simulink model "PassStFwdBkwdCtrl"  (R2018b)
settings: Solver=FixedStepDiscrete  StartTime=0.0  StopTime=10.0  RelTol=1e-3
undefined symbols (not defined in the file or in its folder): KeSMSuMdMotFinshdTm_Val, KeSMSuMdRetryTm1_Val, KeSMSuModeReqDurgTm_Val
libraries: StCtrlLibBkRecln x1
settings Model: ModifiedHistory=2024.6.26 557模式流程V1.6  Creator=sn2xws  LastModifiedBy=sn2xws
settings DataIOCC: SaveFormat=StructureWithTime
settings OptimizationCC: DefaultParameterBehavior=Inlined  EnhancedBackFolding=on  PassReuseOutputArgsAs=Individual arguments  ZeroExternalMemoryAtStartup=off  ZeroInternalMemoryAtStartup=off  OptimizeBlockOrder=speed  DifferentSizesBufferReuse=on  OptimizationCustomize=off
settings DebuggingCC: ParameterTunabilityLossMsg=error
settings SFSimCC: MATLABDynamicMemAlloc=off
settings RTWCC: SystemTargetFile=autosar.tlc  GenCodeOnly=on  TemplateMakefile=ert_default_tmf  Description=AUTOSAR  GenerateReport=on  IncludeHyperlinkInReport=on  LaunchReport=on  GenerateTraceInfo=on  GenerateTraceReport=on  GenerateTraceReportSl=on  GenerateTraceReportSf=on  GenerateTraceReportEml=on
settings CodeAppCC: ForceParamTrailComments=on  IgnoreCustomStorageClasses=off  OperatorAnnotations=on  SimulinkDataObjDesc=on  SFDataObjDesc=on  InsertBlockDesc=on
settings STFCustomTargetCC: TargetLangStandard=C99 (ISO)  MultiwordLength=256  ParMdlRefBuildCompliant=on  CompOptLevelCompliant=on  IncludeMdlTerminateFcn=off  CombineOutputUpdateFcns=on  SuppressErrorStatus=on  ERTCustomFileBanners=on  SupportNonFinite=off  SupportComplex=off  SupportContinuousTime=off  SupportNonInlinedSFcns=off  RemoveResetFunc=on  MATLABClassNameForMDSCustomization=Simulink.SoftwareTarget.ERTCustomization  AutosarCompliant=on  UseToolchainInfoCompliant=on  LookupTableObjectStructAxisOrder=2,1,3,4,...  LUTObjectStructOrderEvenSpacing=Size,Table,Breakpoints  SystemTargetFile=autosar.tlc
settings ERTTargetCC: TargetLangStandard=C99 (ISO)  ConcurrentExecutionCompliant=off  IncludeMdlTerminateFcn=off  SuppressErrorStatus=on  SupportNonFinite=off  SupportComplex=off  ModelStepFunctionPrototypeControlCompliant=off  CPPClassGenCompliant=off  AutosarCompliant=on  LookupTableObjectStructAxisOrder=2,1,3,4,...  LUTObjectStructOrderEvenSpacing=Size,Table,Breakpoints  InlinedParameterPlacement=NonHierarchical  ERTCustomFileTemplate=example_file_process.tlc  ERTFilePackagingFormat=Compact

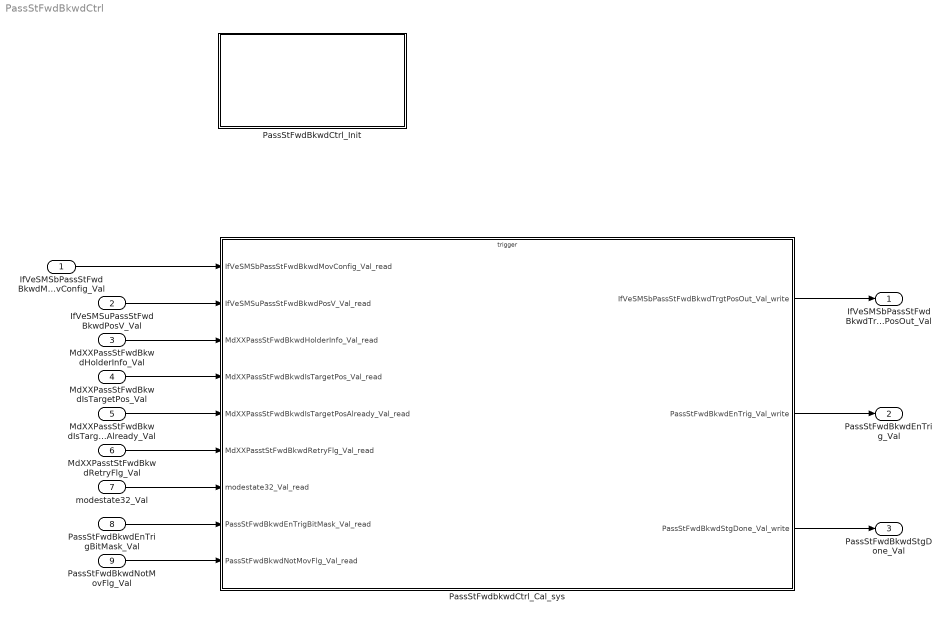
== system PassStFwdBkwdCtrl ==
  IfVeSMSbPassStFwdBkwdMovConfig_Val : Inport  OutDataTypeStr=boolean  PortDimensions=1
  IfVeSMSuPassStFwdBkwdPosV_Val : Inport  Port=2  OutDataTypeStr=boolean  PortDimensions=1
  MdXXPassStFwdBkwdHolderInfo_Val : Inport  Port=3  OutDataTypeStr=uint32  PortDimensions=1
  MdXXPassStFwdBkwdIsTargetPos_Val : Inport  Port=4  OutDataTypeStr=uint32  PortDimensions=1
  MdXXPassStFwdBkwdIsTargetPosAlready_Val : Inport  Port=5  OutDataTypeStr=uint32  PortDimensions=1
  MdXXPasstStFwdBkwdRetryFlg_Val : Inport  Port=6  OutDataTypeStr=uint32  PortDimensions=1
  modestate32_Val : Inport  Port=7  OutDataTypeStr=uint32  PortDimensions=1
  PassStFwdBkwdEnTrigBitMask_Val : Inport  Port=8  OutDataTypeStr=uint32  PortDimensions=1
  PassStFwdBkwdNotMovFlg_Val : Inport  Port=9  OutDataTypeStr=boolean  PortDimensions=1
  PassStFwdBkwdCtrl_Init : Subsystem
  PassStFwdbkwdCtrl_Cal_sys : Subsystem
  IfVeSMSbPassStFwdBkwdTrgtPosOut_Val : Outport  OutDataTypeStr=boolean  PortDimensions=1
  PassStFwdBkwdEnTrig_Val : Outport  Port=2  OutDataTypeStr=boolean  PortDimensions=1
  PassStFwdBkwdStgDone_Val : Outport  Port=3  OutDataTypeStr=boolean  PortDimensions=1
  wires:
  IfVeSMSbPassStFwdBkwdMovConfig_Val/1 -> PassStFwdbkwdCtrl_Cal_sys/1(IfVeSMSbPassStFwdBkwdMovConfig_Val_read)
  IfVeSMSuPassStFwdBkwdPosV_Val/1 -> PassStFwdbkwdCtrl_Cal_sys/2(IfVeSMSuPassStFwdBkwdPosV_Val_read)
  MdXXPassStFwdBkwdHolderInfo_Val/1 -> PassStFwdbkwdCtrl_Cal_sys/3(MdXXPassStFwdBkwdHolderInfo_Val_read)
  MdXXPassStFwdBkwdIsTargetPos_Val/1 -> PassStFwdbkwdCtrl_Cal_sys/4(MdXXPassStFwdBkwdIsTargetPos_Val_read)
  MdXXPassStFwdBkwdIsTargetPosAlready_Val/1 -> PassStFwdbkwdCtrl_Cal_sys/5(MdXXPassStFwdBkwdIsTargetPosAlready_Val_read)
  MdXXPasstStFwdBkwdRetryFlg_Val/1 -> PassStFwdbkwdCtrl_Cal_sys/6(MdXXPasstStFwdBkwdRetryFlg_Val_read)
  modestate32_Val/1 -> PassStFwdbkwdCtrl_Cal_sys/7(modestate32_Val_read)
  PassStFwdBkwdEnTrigBitMask_Val/1 -> PassStFwdbkwdCtrl_Cal_sys/8(PassStFwdBkwdEnTrigBitMask_Val_read)
  PassStFwdBkwdNotMovFlg_Val/1 -> PassStFwdbkwdCtrl_Cal_sys/9(PassStFwdBkwdNotMovFlg_Val_read)
  PassStFwdbkwdCtrl_Cal_sys/1(IfVeSMSbPassStFwdBkwdTrgtPosOut_Val_write) -> IfVeSMSbPassStFwdBkwdTrgtPosOut_Val/1
  PassStFwdbkwdCtrl_Cal_sys/2(PassStFwdBkwdEnTrig_Val_write) -> PassStFwdBkwdEnTrig_Val/1
  PassStFwdbkwdCtrl_Cal_sys/3(PassStFwdBkwdStgDone_Val_write) -> PassStFwdBkwdStgDone_Val/1

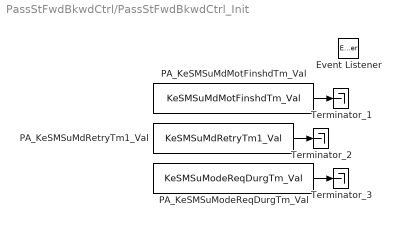
== system PassStFwdBkwdCtrl/PassStFwdBkwdCtrl_Init ==
  Event Listener : EventListener  EventName=reset
  PA_KeSMSuMdMotFinshdTm_Val : Constant  Value=KeSMSuMdMotFinshdTm_Val
  PA_KeSMSuMdRetryTm1_Val : Constant  Value=KeSMSuMdRetryTm1_Val
  PA_KeSMSuModeReqDurgTm_Val : Constant  Value=KeSMSuModeReqDurgTm_Val
  Terminator_1 : Terminator
  Terminator_2 : Terminator
  Terminator_3 : Terminator
  wires:
  PA_KeSMSuMdMotFinshdTm_Val/1 -> Terminator_1/1
  PA_KeSMSuMdRetryTm1_Val/1 -> Terminator_2/1
  PA_KeSMSuModeReqDurgTm_Val/1 -> Terminator_3/1

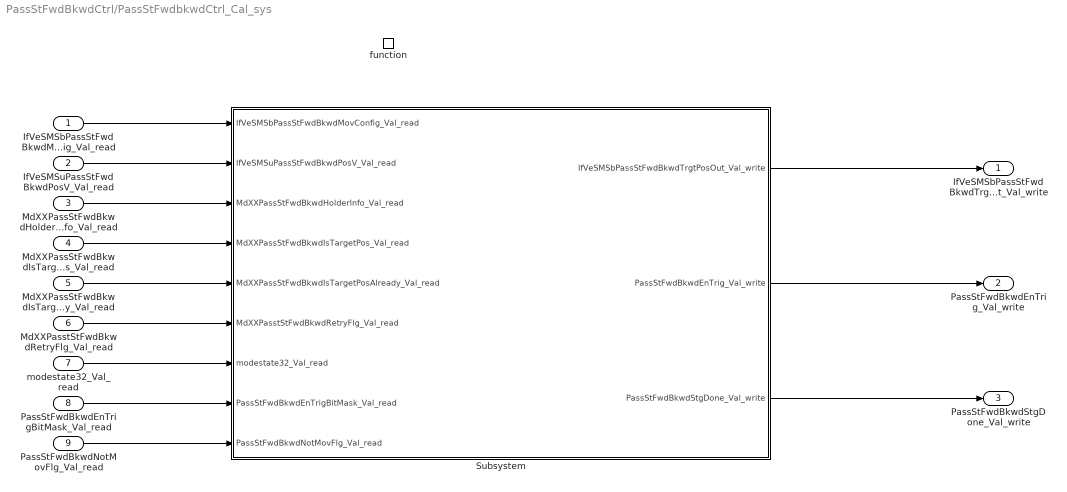
== system PassStFwdBkwdCtrl/PassStFwdbkwdCtrl_Cal_sys ==
  IfVeSMSbPassStFwdBkwdMovConfig_Val_read : Inport
  IfVeSMSuPassStFwdBkwdPosV_Val_read : Inport  Port=2
  MdXXPassStFwdBkwdHolderInfo_Val_read : Inport  Port=3
  MdXXPassStFwdBkwdIsTargetPos_Val_read : Inport  Port=4
  MdXXPassStFwdBkwdIsTargetPosAlready_Val_read : Inport  Port=5
  MdXXPasstStFwdBkwdRetryFlg_Val_read : Inport  Port=6
  modestate32_Val_read : Inport  Port=7
  PassStFwdBkwdEnTrigBitMask_Val_read : Inport  Port=8
  PassStFwdBkwdNotMovFlg_Val_read : Inport  Port=9
  function : TriggerPort  TriggerType=function-call  IsSimulinkFunction=on  FunctionName=PassStFwdbkwdCtrl_Cal  VariantControl=(inherit)
  Subsystem : Subsystem
  IfVeSMSbPassStFwdBkwdTrgtPosOut_Val_write : Outport
      settings: EnsureOutportIsVirtual=on
  PassStFwdBkwdEnTrig_Val_write : Outport  Port=2
      settings: EnsureOutportIsVirtual=on
  PassStFwdBkwdStgDone_Val_write : Outport  Port=3
      settings: EnsureOutportIsVirtual=on
  wires:
  IfVeSMSbPassStFwdBkwdMovConfig_Val_read/1 -> Subsystem/1(IfVeSMSbPassStFwdBkwdMovConfig_Val_read)
  IfVeSMSuPassStFwdBkwdPosV_Val_read/1 -> Subsystem/2(IfVeSMSuPassStFwdBkwdPosV_Val_read)
  MdXXPassStFwdBkwdHolderInfo_Val_read/1 -> Subsystem/3(MdXXPassStFwdBkwdHolderInfo_Val_read)
  MdXXPassStFwdBkwdIsTargetPos_Val_read/1 -> Subsystem/4(MdXXPassStFwdBkwdIsTargetPos_Val_read)
  MdXXPassStFwdBkwdIsTargetPosAlready_Val_read/1 -> Subsystem/5(MdXXPassStFwdBkwdIsTargetPosAlready_Val_read)
  MdXXPasstStFwdBkwdRetryFlg_Val_read/1 -> Subsystem/6(MdXXPasstStFwdBkwdRetryFlg_Val_read)
  modestate32_Val_read/1 -> Subsystem/7(modestate32_Val_read)
  PassStFwdBkwdEnTrigBitMask_Val_read/1 -> Subsystem/8(PassStFwdBkwdEnTrigBitMask_Val_read)
  PassStFwdBkwdNotMovFlg_Val_read/1 -> Subsystem/9(PassStFwdBkwdNotMovFlg_Val_read)
  Subsystem/1(IfVeSMSbPassStFwdBkwdTrgtPosOut_Val_write) -> IfVeSMSbPassStFwdBkwdTrgtPosOut_Val_write/1
  Subsystem/2(PassStFwdBkwdEnTrig_Val_write) -> PassStFwdBkwdEnTrig_Val_write/1
  Subsystem/3(PassStFwdBkwdStgDone_Val_write) -> PassStFwdBkwdStgDone_Val_write/1

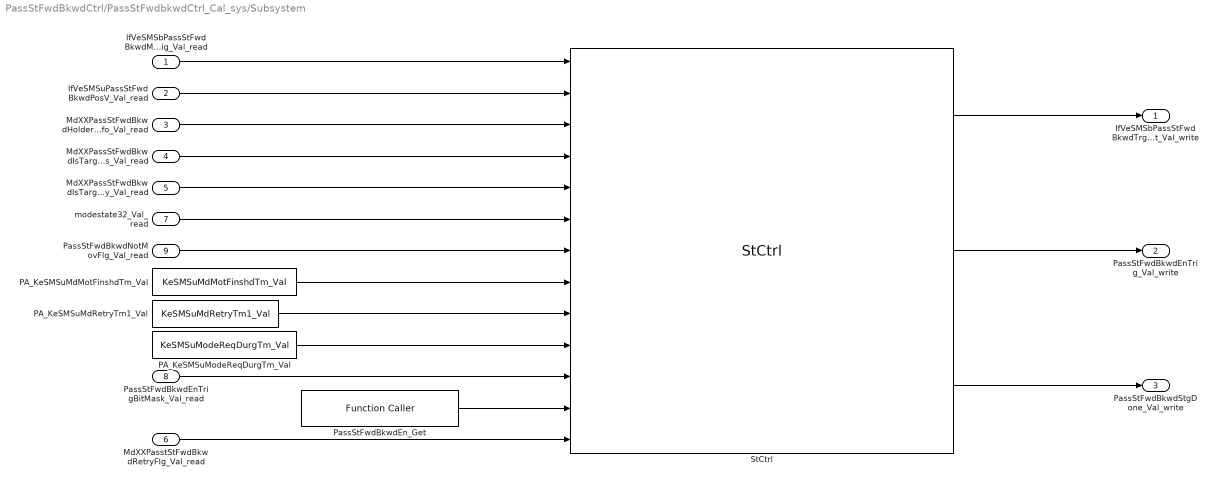
== system PassStFwdBkwdCtrl/PassStFwdbkwdCtrl_Cal_sys/Subsystem ==
  IfVeSMSbPassStFwdBkwdMovConfig_Val_read : Inport
  IfVeSMSuPassStFwdBkwdPosV_Val_read : Inport  Port=2
  MdXXPassStFwdBkwdHolderInfo_Val_read : Inport  Port=3
  MdXXPassStFwdBkwdIsTargetPos_Val_read : Inport  Port=4
  MdXXPassStFwdBkwdIsTargetPosAlready_Val_read : Inport  Port=5
  MdXXPasstStFwdBkwdRetryFlg_Val_read : Inport  Port=6
  modestate32_Val_read : Inport  Port=7
  PassStFwdBkwdEnTrigBitMask_Val_read : Inport  Port=8
  PassStFwdBkwdNotMovFlg_Val_read : Inport  Port=9
  PA_KeSMSuMdMotFinshdTm_Val : Constant  Value=KeSMSuMdMotFinshdTm_Val
  PA_KeSMSuMdRetryTm1_Val : Constant  Value=KeSMSuMdRetryTm1_Val
  PA_KeSMSuModeReqDurgTm_Val : Constant  Value=KeSMSuModeReqDurgTm_Val
  PassStFwdBkwdEn_Get : FunctionCaller  FunctionPrototype=data = PassStFwdBkwdEn_Get()  OutputArgumentSpecifications=uint32(1)
  StCtrl : StCtrlLibBkRecln/StCtrl  SystemSampleTime=-1
  IfVeSMSbPassStFwdBkwdTrgtPosOut_Val_write : Outport
      settings: EnsureOutportIsVirtual=on
  PassStFwdBkwdEnTrig_Val_write : Outport  Port=2
      settings: EnsureOutportIsVirtual=on
  PassStFwdBkwdStgDone_Val_write : Outport  Port=3
      settings: EnsureOutportIsVirtual=on
  wires:
  PA_KeSMSuModeReqDurgTm_Val/1 -> StCtrl/10
  PassStFwdBkwdEn_Get/1 -> StCtrl/12
  StCtrl/3 -> PassStFwdBkwdStgDone_Val_write/1
  StCtrl/2 -> PassStFwdBkwdEnTrig_Val_write/1
  StCtrl/1 -> IfVeSMSbPassStFwdBkwdTrgtPosOut_Val_write/1
  IfVeSMSbPassStFwdBkwdMovConfig_Val_read/1 -> StCtrl/1
  IfVeSMSuPassStFwdBkwdPosV_Val_read/1 -> StCtrl/2
  MdXXPassStFwdBkwdHolderInfo_Val_read/1 -> StCtrl/3
  MdXXPassStFwdBkwdIsTargetPos_Val_read/1 -> StCtrl/4
  MdXXPassStFwdBkwdIsTargetPosAlready_Val_read/1 -> StCtrl/5
  modestate32_Val_read/1 -> StCtrl/6
  PassStFwdBkwdNotMovFlg_Val_read/1 -> StCtrl/7
  PA_KeSMSuMdMotFinshdTm_Val/1 -> StCtrl/8
  PA_KeSMSuMdRetryTm1_Val/1 -> StCtrl/9
  PassStFwdBkwdEnTrigBitMask_Val_read/1 -> StCtrl/11
  MdXXPasstStFwdBkwdRetryFlg_Val_read/1 -> StCtrl/13
